simulink model "BlockDemo"  (Simulink 6.3)
settings: Solver=ode45  StartTime=0.0  StopTime=10.0  RelTol=1e-3
InitFcn:
  | %% DSPBuilder Start
  | alt_dspbuilder_update_model(bdroot)
  | %% DSPBuilder End
libraries: allblocks_alteradspbuilder2 x6
settings Model: LastModifiedBy=delphick
settings OptimizationCC: BooleanDataType=off  InlineInvariantSignals=on
settings DebuggingCC: SolverPrmCheckMsg=none
settings HardwareCC: TargetUnknown=on

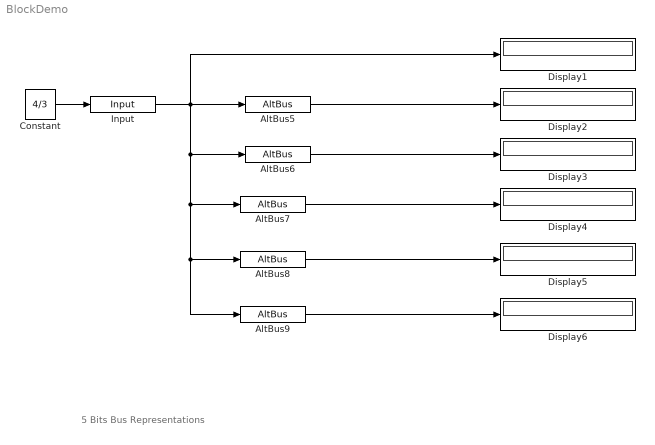
== system BlockDemo ==
  note: 5 Bits Bus Representations
  AltBus5 : allblocks_alteradspbuilder2/AltBus  BusType=Signed Fractional  bwl=5  bwr=0  saturate=off
  AltBus6 : allblocks_alteradspbuilder2/AltBus  BusType=Signed Fractional  bwl=4  bwr=1  saturate=off
  AltBus7 : allblocks_alteradspbuilder2/AltBus  BusType=Signed Fractional  bwl=3  bwr=2  saturate=off
  AltBus8 : allblocks_alteradspbuilder2/AltBus  BusType=Signed Fractional  bwl=2  bwr=3  saturate=off
  AltBus9 : allblocks_alteradspbuilder2/AltBus  BusType=Signed Fractional  bwl=1  bwr=4  saturate=off
  Constant : Constant  Value=4/3
  Display{1..6} (6 alike) : Display
  Input : allblocks_alteradspbuilder2/Input  iofile=C:\workspace_clean\Documentation\DesignExamples\Tutorials\UnitBlocks\IOBus\AltBus\tb_BlockDemo\BlockDemo_Input.salt  BusType=Signed Fractional  bwl=10  bwr=10  SpecifyClock=off  PORTTYPE=Input
  wires:
  Constant/1 -> Input/1
  AltBus5/1 -> Display2/1
  AltBus6/1 -> Display3/1
  AltBus7/1 -> Display4/1
  AltBus8/1 -> Display5/1
  AltBus9/1 -> Display6/1
  Input/1 -> AltBus8/1, AltBus9/1, AltBus7/1, AltBus6/1, Display1/1, AltBus5/1
